simulink model "FLCSim"  (R2019a)
settings: Solver=VariableStepAuto  StartTime=0.0  StopTime=5  MaxStep=0.01  RelTol=1e-4  EnableMultiTasking=on
libraries: fuzblock x1
settings Model: Creator=Nikos  LastModifiedBy=gitop
settings DataIOCC: LimitDataPoints=on  SaveOutput=off  SaveTime=off  ReturnWorkspaceOutputs=off
settings OptimizationCC: ExpressionDepthLimit=2147483647  LifeSpan=1
settings DebuggingCC: UnderspecifiedInitializationDetection=Classic  MergeDetectMultiDrivingBlocksExec=none  FcnCallInpInsideContextMsg=warning  AllowSymbolicDim=off  StateNameClashWarn=warning  PregeneratedLibrarySubsystemCodeDiagnostic=none  SFUnexpectedBacktrackingDiag=warning  SFNoUnconditionalDefaultTransitionDiag=warning  SFExecutionAtInitializationDiag=none  ArithmeticOperatorsInVariantConditions=warning
settings SFSimCC: SimUseLocalCustomCode=off
settings RTWCC: RTWUseLocalCustomCode=off
settings CodeAppCC: StateflowObjectComments=on
settings GRTTargetCC: TargetLangStandard=C89/C90 (ANSI)  GeneratePreprocessorConditionals=Disable all  CombineOutputUpdateFcns=off  GRTInterface=on

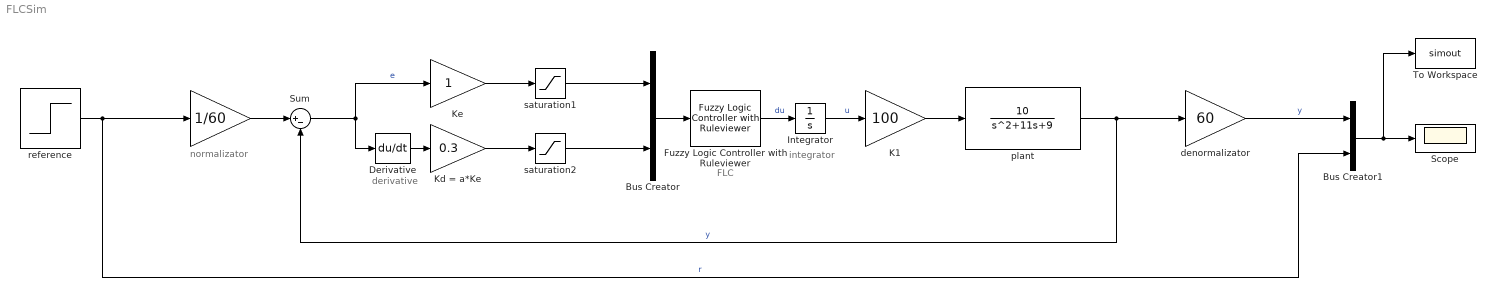
== system FLCSim ==
  note: FLC
  note: derivative
  note: integrator
  note: normalizator
  " " : Gain  Gain=1/60
  " denormalizator" : Gain  Gain=60
  " Κ1" : Gain  Gain=100
  Bus Creator : BusCreator  Inputs=2
  Bus Creator1 : BusCreator  Inputs=2
  Derivative : Derivative
  Fuzzy Logic Controller with Ruleviewer : fuzblock/Fuzzy Logic  Controller  with Ruleviewer  fismatrix=FLC  Ts=.1
  Integrator : Integrator
  Kd = a*Ke : Gain  Gain=0.3
  Ke : Gain
  Scope : Scope
  Sum : Sum  Inputs=|+-
  To Workspace : ToWorkspace  VariableName=simout  SaveFormat=Structure With Time  SampleTime=-1
  plant : TransferFcn  Numerator=[10]  Denominator=[1 11 9]
  reference : Step  Time=0.1  After=60  SampleTime=0.01
  saturation1 : Saturate  UpperLimit=0.99  LowerLimit=-0.99
  saturation2 : Saturate  UpperLimit=0.99  LowerLimit=-0.99
  wires:
  plant/1 -> " denormalizator"/1, Sum/2  "y"
  reference/1 -> Bus Creator1/2, " "/1  "r"
  Fuzzy Logic Controller with Ruleviewer/1 -> Integrator/1  "du"
  Bus Creator/1 -> Fuzzy Logic Controller with Ruleviewer/1
  Ke/1 -> saturation1/1
  Sum/1 -> Derivative/1, Ke/1  "e"
  Derivative/1 -> Kd = a*Ke/1
  saturation2/1 -> Bus Creator/2
  " "/1 -> Sum/1
  Integrator/1 -> " Κ1"/1  "u"
  saturation1/1 -> Bus Creator/1
  Kd = a*Ke/1 -> saturation2/1
  " denormalizator"/1 -> Bus Creator1/1  "y"
  " Κ1"/1 -> plant/1
  Bus Creator1/1 -> To Workspace/1, Scope/1
